simulink model "rev0BB"  (R2017b)
settings: Solver=FixedStepDiscrete  StartTime=0  StopTime=(((preLen+100+dataLenSymbols)*1+pad_first*3)*basePer)  RelTol=1e-3
values from neighbouring files (symbols this model uses):
  ack_stf_len_symbols = length(x_ACK_STF)    [rev0BB_setup.m]
  agc_delay_lag = 32    [rev0BB_setup.m]
  agc_detector_coef = ones(1,agc_detector_taps)./agc_detector_taps    [rev0BB_setup.m]
  agc_on = true    [rev0BB_startup.m]
  agc_sat_low = -agcSaturation    (= -12)    [rev0BB_setup.m]
  agc_sat_up = agcSaturation    (= 12)    [rev0BB_setup.m]
  agcDesired = 0    [rev0BB_setup.m]
  agcExpDomain = agcSaturation    (= 12)    [rev0BB_setup.m]
  agcExpResolution = 2^-5    (= 0.03125)    [rev0BB_setup.m]
  agcPwrAvgNum = 128    [rev0BB_setup.m]
  agcSaturation = 12    [rev0BB_setup.m]
  agcSettleThresh = 0.65    [rev0BB_setup.m]
  agcStep = 2^-8    (= 0.00390625)    [rev0BB_setup.m]
  atanDomain = 5    [rev0BB_setup.m]
  atanDomainTiming = 256    [rev0BB_setup.m]
  atanResolution = 2^-9    (= 0.001953125)    [rev0BB_setup.m]
  atanResolutionTiming = 2^-5    (= 0.03125)    [rev0BB_setup.m]
  averaging_num = ones(1, averaging_samples)    [rev0BB_setup.m]
  averaging_samples = 128    [rev0BB_setup.m]
  awgnSeed = abs(dBSnrRange(dBSnrInd)*1000+trial+10000000)    [plotBer.m]    (also in rev0BB_startup.m = 67)
  basePer = 1/baseFreq    (= 5e-08)    [rev0BB_setup.m]
  bitsPerSymbolHeader = log2(radixHeader)    [rev0BB_setup.m]
  bitsPerSymbolMax = log2(radixMax)    [rev0BB_setup.m]
  cal_sig_i_mult = 1.0    (= 1)    [rev0BB_startup.m]
  cal_sig_i_offset = 0.0    (= 0)    [rev0BB_startup.m]
  cal_sig_q_mult = 1.0    (= 1)    [rev0BB_startup.m]
  cal_sig_q_offset = 0.0    (= 0)    [rev0BB_startup.m]
  cefEarlyWarning = 256    [rev0BB_setup.m]
  cefLen = length(x_CEF)    [rev0BB_setup.m]
  channelFIR = zeros(1, round(maxSampleDelay)+1)    [rev0BB_startup.m]
  coarseCFOAdaptDelay = 1    [rev0BB_setup.m]
  cr_i = 0.020    (= 0.02)    [rev0BB_setup.m]
  cr_i_preamp = 2^-9    (= 0.001953125)    [rev0BB_setup.m]
  cr_int1_sat_low = -cr_integrator1_saturation    (= -0.6)    [rev0BB_setup.m]
  cr_int1_sat_up = cr_integrator1_saturation    (= 0.6)    [rev0BB_setup.m]
  cr_integrator1_decay = 1    [rev0BB_setup.m]
  cr_integrator1_saturation = 0.6    [rev0BB_setup.m]
  cr_mult_pipeline = 0    [rev0BB_setup.m]
  cr_p = 0.015    [rev0BB_setup.m]
  cr_sat2_low = -cr_saturation2    (= -0.6)    [rev0BB_setup.m]
  cr_sat2_up = cr_saturation2    (= 0.6)    [rev0BB_setup.m]
  cr_smooth_num = (1/cr_smooth_samples).*ones(1, cr_smooth_samples)    [rev0BB_setup.m]
  D_128 = [ 1,  8,  2,  4, 16, 32, 64]    [golay.m]    (also in rev0BB_setup.m)
  D_32 = [ 1,  4,  8,  2, 16]    [golay.m]    (also in rev0BB_setup.m)
  dataLenSymbols = header_len_bytes*8/bitsPerSymbolHeader + frame_len_bytes*8/bitsPerSymbol    [rev0BB_setup.m]
  default_channel = 3    [rev0BB_setup.m]
  dmm_coefs = ones(1,dmm_samples)./dmm_samples    [rev0BB_setup.m]
  dst_field_len = 8    [rev0BB_setup.m]
  expDomain = 3.3    [rev0BB_setup.m]
  expResolution = 2^-5    (= 0.03125)    [rev0BB_setup.m]
  expTol = .1    (= 0.1)    [rev0BB_setup.m]
  flush_delay = regular_pipeline*2+mult_pipeline+4    (= 4)    [rev0BB_setup.m]
  frac_lut_domain = 256    [rev0BB_setup.m]
  frac_lut_domain_cr = 64    [rev0BB_setup.m]
  frac_lut_range_max = 512    [rev0BB_setup.m]
  frac_lut_range_max_coarse_cfo = 127    [rev0BB_setup.m]
  frac_lut_range_max_cr = 127    [rev0BB_setup.m]
  frac_lut_range_min = -frac_lut_range_max    (= -512)    [rev0BB_setup.m]
  frac_lut_range_min_coarse_cfo = -frac_lut_range_max_coarse_cfo    (= -127)    [rev0BB_setup.m]
  frac_lut_range_min_cr = -frac_lut_range_max_cr    (= -127)    [rev0BB_setup.m]
  frac_lut_table_breaks = -frac_lut_domain:frac_lut_res:(frac_lut_domain-1)    [rev0BB_setup.m]
  frac_lut_table_breaks_coarse_cfo = -frac_lut_domain_coarse_cfo:frac_lut_res_coarse_cfo:(frac_lut_domain_coarse_cfo-1)    [rev0BB_setup.m]
  frac_lut_table_breaks_cr = -frac_lut_domain_cr:frac_lut_res_cr:(frac_lut_domain_cr-1)    [rev0BB_setup.m]
  frac_lut_table_data = 1./frac_lut_table_breaks    [rev0BB_setup.m]
  frac_lut_table_data_coarse_cfo = 1./frac_lut_table_breaks_coarse_cfo    [rev0BB_setup.m]
  frac_lut_table_data_cr = 1./frac_lut_table_breaks_cr    [rev0BB_setup.m]
  freeze_en_agc = true    [rev0BB_startup.m]
  freeze_en_cr_int1 = false    [rev0BB_startup.m]
  freeze_en_cr_int2 = false    [rev0BB_startup.m]
  freeze_en_cr_phase = false    [rev0BB_startup.m]
  freeze_en_tr_int1 = false    [rev0BB_startup.m]
  freeze_en_tr_int2 = false    [rev0BB_startup.m]
  freeze_en_tr_phase = false    [rev0BB_startup.m]
  freeze_on_cef_done = true    [rev0BB_startup.m]
  freeze_on_stf_done = false    [rev0BB_startup.m]
  freeze_on_valid = true    [rev0BB_startup.m]
  golay_type = 32    [rev0BB_setup.m]
  guardInt = int16(4)    [rev0BB_setup.m]
  guardTol = int16(5)    [rev0BB_setup.m]
  header_len_bytes = 8    [rev0BB_setup.m]
  lineWidth = 60    [rev0BB_setup.m]
  lmsEqDepth = 38    [rev0BB_setup.m]
  lmsStep_init = 0.006    [rev0BB_setup.m]
  lmsStep_meta = (lmsStep_final - lmsStep_init)/cefLen    [rev0BB_setup.m]
  lnDomain = 16    [rev0BB_setup.m]
  lnResolution = 2^-5    (= 0.03125)    [rev0BB_setup.m]
  local_node_id = 2    [rev0BB_startup.m]
  maxMsgSize = length(xSpectrum_PRE)+dataLenSymbols+300    [rev0BB_setup.m]
  minSTFPeaks = 3    [rev0BB_setup.m]
  mod_scheme_len_bytes = 1    [rev0BB_setup.m]
  modBPS = [1, 2, 4]    [rev0BB_setup.m]
  modKeys = [0, 1, 2]    [rev0BB_setup.m]
  mult_pipeline = 0    [rev0BB_setup.m]
  overSampleFreq = 80e6    (= 80000000)    [rev0BB_setup.m]
  overSamplePer = 1/overSampleFreq    (= 1.25e-08)    [rev0BB_setup.m]
  pad_first = 1000    [createTestVectors.m]
  post_cr_i_offset = 0    [rev0BB_startup.m]
  post_cr_q_offset = 0    [rev0BB_startup.m]
  preambleSequentialDetect = 2    [rev0BB_setup.m]
  preLen = length(x_PRE)    [rev0BB_setup.m]
  qam16_demod_scale_factor = qam16_hdl_distance/qam16_power_normalized_distance    [rev0BB_setup.m]
  rcRxFilt = [0.000303163120401141 -0.00118915940834234 -0.00187387637177 -0.00124167532697737 0.00029186889076529 0.00164526160586517 0.00182432050803312 0.000652133621739543 -0.00105668254004908 -0.00204011570659167 -0.00150058088768918 0.00026138356356816 0.0019831869994874 0.00231075800085521 0.000821993419120097 -0.00154687337975486 -0.00305430783933469 -0.00238186490079127 0.000301216962040692 0.00325307 ...(+2001 chars)    [rev0BB_setup.m]
  rcTxFilt = [0.000303163120401141 -0.00118915940834234 -0.00187387637177 -0.00124167532697737 0.00029186889076529 0.00164526160586517 0.00182432050803312 0.000652133621739543 -0.00105668254004908 -0.00204011570659167 -0.00150058088768918 0.00026138356356816 0.0019831869994874 0.00231075800085521 0.000821993419120097 -0.00154687337975486 -0.00305430783933469 -0.00238186490079127 0.000301216962040692 0.00325307 ...(+2001 chars)    [rev0BB_setup.m]
  regular_pipeline = 0    [rev0BB_setup.m]
  rx_gain = 1    [rev0BB_setup.m]
  rx_gain_i = 1    [rev0BB_setup.m]
  rx_gain_q = 1    [rev0BB_setup.m]
  rx_impare_i_offset = 0    [rev0BB_startup.m]
  rx_impare_i_scale = 1    [rev0BB_startup.m]
  rx_impare_q_offset = 0    [rev0BB_startup.m]
  rx_impare_q_scale = 1    [rev0BB_startup.m]
  rx_offset_correction_i = 0    [rev0BB_startup.m]
  rx_offset_correction_q = 0    [rev0BB_startup.m]
  sin_source_amp = 1    [rev0BB_setup.m]
  sin_source_freq = 250e6/16    (= 15625000)    [rev0BB_setup.m]
  slowPer = overSamplePer*slowSample    (= 2.5e-08)    [rev0BB_setup.m]
  std_pkt_type = 0    [rev0BB_setup.m]
  stfLen = length(x_STF)    [rev0BB_setup.m]
  testMsg = cat(1, xCTRL_PRE_adj, header, payload)    [plotBer.m]
  timing_i = 0.25    [rev0BB_setup.m]
  ... (+25 more)
undefined symbols (not defined in the file or in its folder): cr_integrator2_saturation, doppler, i, magnitude, useFadingChannel
libraries: helperLib x128, simulink x90, golayLib x34, dspsigops x32, commfilt2 x27, commdigbbndpm3 x8, hdlsllib x6, dsparch4 x4, commdigbbndam3 x4, commchan3 x2, commrflib2 x2, commcrc2 x2
(part 1 of 10)
settings Model: FPTRunName=FPA_Reference  ExtModeTrigDuration=100  Creator=cyarp  LastModifiedBy=cyarp
settings SolverCC: InsertRTBMode=Always
settings DataIOCC: LimitDataPoints=on  SaveFinalState=on  SaveFormat=StructureWithTime  SaveOutput=off  SaveState=on  StateSaveName=tmp_raccel_xout  SignalLoggingName=tmp_raccel_logsout
settings OptimizationCC: DefaultParameterBehavior=Inlined  UseDivisionForNetSlopeComputation=on  UseFloatMulNetSlope=on  InlineInvariantSignals=on  PassReuseOutputArgsAs=Individual arguments  EfficientFloat2IntCast=on  SimCompilerOptimization=on  OptimizeBlockOrder=speed  DifferentSizesBufferReuse=on
settings DebuggingCC: AlgebraicLoopMsg=error  SolverPrmCheckMsg=warning  SingleTaskRateTransMsg=error  ParameterTunabilityLossMsg=error  SFUnexpectedBacktrackingDiag=warning  SFNoUnconditionalDefaultTransitionDiag=warning  SFExecutionAtInitializationDiag=none
settings HardwareCC: ProdBitPerLong=64  ProdHWDeviceType=Intel->x86-64 (Linux 64)  TargetBitPerLong=64  TargetBitPerPointer=64  TargetBitPerSizeT=64  TargetBitPerPtrDiffT=64  TargetLongLongMode=on  TargetIntDivRoundTo=Zero  TargetEndianess=LittleEndian  TargetWordSize=64  TargetHWDeviceType=MATLAB Host
settings ModelReferenceCC: PropagateSignalLabelsOutOfModel=off
settings SFSimCC: MATLABDynamicMemAlloc=off
settings RTWCC: SystemTargetFile=ert.tlc  TemplateMakefile=ert_default_tmf  GenerateReport=on  SaveLog=on  RTWUseSimCustomCode=on  BuildConfiguration=Faster Runs  IncludeHyperlinkInReport=on  LaunchReport=on  CreateSILPILBlock=SIL  GenerateTraceInfo=on  GenerateTraceReport=on  GenerateTraceReportSl=on  GenerateTraceReportSf=on  GenerateTraceReportEml=on  GenerateCodeMetricsReport=on  GenerateCodeReplacementReport=on
settings CodeAppCC: ForceParamTrailComments=on  IgnoreCustomStorageClasses=off  OperatorAnnotations=on  SimulinkDataObjDesc=on  SFDataObjDesc=on  InsertBlockDesc=on
settings ERTTargetCC: TargetLangStandard=C99 (ISO)  GenerateSampleERTMain=on  ERTCustomFileTemplate=example_file_process.tlc
settings ConfigComp: CovScope=Subsystem  CovPath=receiver  CovMetricSettings=dw  CovHtmlReporting=on  CovSaveCumulativeToWorkspaceVar=on  CovSaveSingleToWorkspaceVar=on  CovExternalEMLEnable=off  CovSFcnEnable=off
settings SimscapeCC: SimscapeNormalizeSystem=off

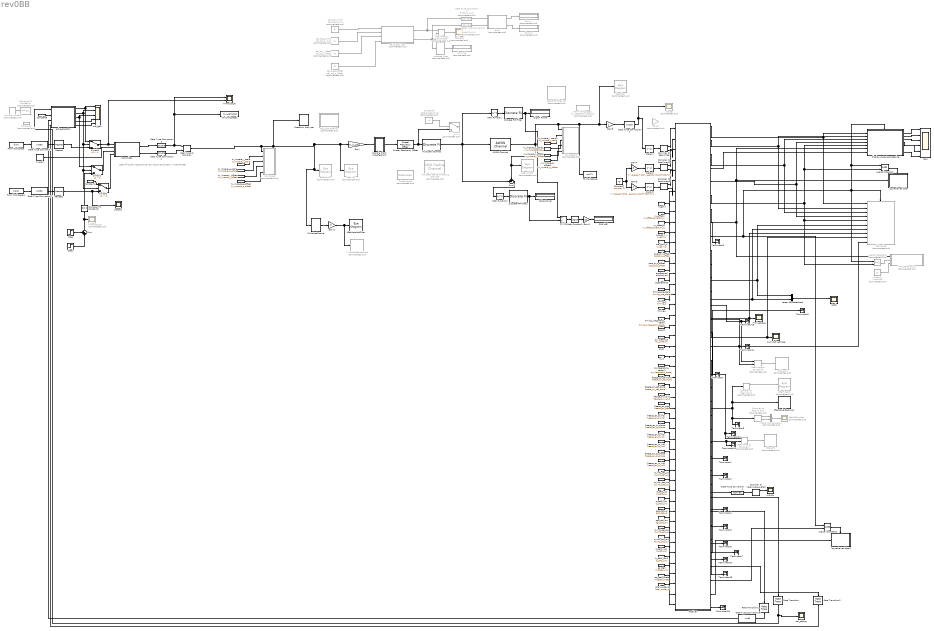
== system rev0BB ==
  note: Zero filling for upsampling now occurs explicitally in transmitter
  " AfterAGC" : ConstellationDiagram  Commented=on
  " AfterCarrierRecovery" : ConstellationDiagram
  ADC_DAC Filtering : Subsystem  Commented=on
  ADC_DAC Filtering1 : Subsystem  Commented=on
  AWGN Channel : commchan3/AWGN Channel  InputProcessing=Columns as channels (frame based)  seed=awgnSeed  noiseMode="Signal to noise ratio  (SNR)"  EbNodB=awgnEbN0  EsNodB=10  SNRdB=awgnSNR  bitsPerSym=1  Ps=1  Tsym=basePer  variance=1
  After AWGN : EyeDiagram  Commented=on
  After LPF : EyeDiagram  Commented=on
  AfterChan : EyeDiagram  Commented=on
  AfterCrSamples : Scope  Commented=on
  AfterFineCR : EyeDiagram  Commented=on
  AfterMatchedFilter : EyeDiagram
  Before LPF : EyeDiagram  Commented=on
  CaCb : Scope  NumInputPorts=3
  CalSignal : Scope  Commented=on
  Compare To Constant1 : simulink/Logic and Bit Operations/Compare To Constant  Commented=on  relop===  const=511  OutDataTypeStr=boolean
  Compare To Constant2 : simulink/Logic and Bit Operations/Compare To Constant  relop===  const=0  OutDataTypeStr=boolean
  Complex to Magnitude-Angle2 : ComplexToMagnitudeAngle
  Complex to Real-Imag : ComplexToRealImag
  Complex to Real-Imag1 : ComplexToRealImag
  Complex to Real-Imag2 : ComplexToRealImag  Commented=on
  Complex to Real-Imag3 : ComplexToRealImag
  Complex to Real-Imag4 : ComplexToRealImag  Commented=on
  Constant : Constant  Commented=on  Value=lineWidth
  Constant2 : Constant  Value=complex(0)  OutDataTypeStr=Inherit: Inherit via back propagation  SampleTime=-1
  Constant3 : Constant  Commented=on  Value=useFadingChannel  OutDataTypeStr=boolean
  Constant4 : Constant  Value=0  OutDataTypeStr=uint32  SampleTime=-1
  Constant5 : Constant  Value=false  OutDataTypeStr=Inherit: Inherit via back propagation  SampleTime=-1
  Constant6 : Constant  Commented=on  Value=5  OutDataTypeStr=Inherit: Inherit via back propagation  SampleTime=-1
  Counter Limited : simulink/Sources/Counter Limited  Commented=on  uplimit=511  tsamp=-1
  CumulativePhase : Scope
  Data Type Conversion : DataTypeConversion  OutDataTypeStr=uint32  RndMeth=Nearest
  Data Type Conversion1 : DataTypeConversion  OutDataTypeStr=single
  Data Type Conversion2 : DataTypeConversion  OutDataTypeStr=double  RndMeth=Nearest
  Data Type Conversion3 : DataTypeConversion  OutDataTypeStr=double  RndMeth=Nearest
  Data Type Conversion4 : DataTypeConversion
  Data Type Conversion5 : DataTypeConversion  Commented=on  OutDataTypeStr=fixdt(1,14,11)
  Data Type Conversion6 : DataTypeConversion  Commented=on  OutDataTypeStr=fixdt(1,14,11)
  Data Type Conversion7 : DataTypeConversion  OutDataTypeStr=uint32  RndMeth=Nearest
  Data Type Conversion9 : DataTypeConversion  OutDataTypeStr=uint8
  Delay1 : Delay  DelayLength=3  InitialCondition=0
  Delay2 : Delay  DelayLength=(preLen+100+dataLenSymbols+100)*4*2  InitialCondition=0
  Delay3 : Delay  DelayLength=(preLen+100+dataLenSymbols+100)*4*1  InitialCondition=0
  Discrete FIR Filter : DiscreteFir  Coefficients=ones(1,10000)./10000  InputProcessing=Columns as channels (frame based)
  Discrete FIR Filter1 : DiscreteFir  Coefficients=ones(1,10000)./10000  InputProcessing=Columns as channels (frame based)
  Divide : Product  Inputs=*/
  FSM : Scope  NumInputPorts=6
  From Workspace : FromWorkspace  VariableName=simX  SampleTime=basePer*1  Interpolate=off  OutputAfterFinalValue=Setting to zero
  From Workspace1 : FromWorkspace  VariableName=modX  SampleTime=basePer*1  Interpolate=off  OutputAfterFinalValue=Setting to zero
  From Workspace2 : FromWorkspace  Commented=on  VariableName=tx_integration_test_sig  SampleTime=overSamplePer*1  Interpolate=off  OutputAfterFinalValue=Setting to zero
  Gain : Gain  Gain=tx_rx_gain
  Gain1 : Gain  Gain=10
  Gain2 : Gain  Gain=.5
  Gain3 : Gain
  Gain4 : Gain  Gain=.5  OutDataTypeStr=Inherit: Same as input
  Gain5 : Gain  Gain=.1  OutDataTypeStr=Inherit: Same as input
  Gain6 : Gain  Commented=on  Gain=.001  OutDataTypeStr=Inherit: Same as input
  IQ_Impare : Subsystem  Commented=on
  IQ_Impare1 : Subsystem  Commented=on
  LMS Err : Scope
  Logical Operator : Logic  AllPortsSameDT=off  OutDataTypeStr=boolean
  Logical Operator1 : Logic  Commented=on  AllPortsSameDT=off  OutDataTypeStr=boolean
  Logical Operator2 : Logic  AllPortsSameDT=off  OutDataTypeStr=boolean
  MATLAB Function : MATLAB Function  Commented=on  TreatAsAtomicUnit=on
  Math Function : Math  Operator=magnitude^2  OutputSignalType=real  SaturateOnIntegerOverflow=on
  Math Function1 : Math  Operator=magnitude^2  OutputSignalType=real  SaturateOnIntegerOverflow=on
  Math Function2 : Math  Operator=log10  OutputSignalType=real  SaturateOnIntegerOverflow=on
  Multipath Channel : DiscreteFir  Coefficients=channelFIR  InputProcessing=Columns as channels (frame based)
  Multipath Rayleigh Fading Channel : commchan3/SISO Fading Channel  Commented=on  PathDelays=chanDelays  AveragePathGains=chanPathGains  NormalizePathGains=on  FadingDistribution=Rayleigh  KFactor=3  DirectPathDopplerShift=0  DirectPathInitialPhase=0  MaximumDopplerShift=maxDopplerHz  DopplerSpectrum=doppler('Flat')  RandomStream=mt19937ar with seed  RandomNumGenerator=shr3cong  Seed=awgnSeed  PathGainsOutputPort=on  ChannelFilterDelayOutputPort=on  SimulateUsing=Interpreted execution  Visualization=Off  PathsForDopplerDisplay=1  SamplesToDisplay=25%
      settings: SourceProductName=Communications System Toolbox
  Noise Power : Display
  Origional : ConstellationDiagram  Commented=on
  Phase Noise : commrflib2/Phase Noise  Commented=on  PhNs=-100  Fo=10000  Fs=overSampleFreq  seed=2137
      settings: SourceProductName=Communications System Toolbox  SourceProductBaseCode=CM
  Phase/ Frequency Offset : commrflib2/Phase// Frequency Offset  phaseOffset=rxPhaseOffset  freqPort=off  freqOffset=freqOffsetHz
      settings: SourceProductName=Communications System Toolbox
  Rate Transition : RateTransition
  Rate Transition1 : RateTransition
  Rate Transition2 : RateTransition
  Real-Imag to Complex : RealImagToComplex
  Real-Imag to Complex2 : RealImagToComplex  Commented=on
  Real-Imag to Complex3 : RealImagToComplex  Commented=on
  Real-Imag to Complex6 : RealImagToComplex  Commented=on
  Repeat : dspsigops/Repeat  N=4  RateOptions=Allow multirate processing  ic=0  mode=Unused parameter value
      settings: SourceProductName=DSP System Toolbox
  Repeat1 : dspsigops/Repeat  N=4  RateOptions=Allow multirate processing  ic=0  mode=Unused parameter value
      settings: SourceProductName=DSP System Toolbox
  RxRaisedCosine : Subsystem
  SNR (dB) : Display
  Sample Clock Imperfections : Subsystem
  Scope : Scope  Commented=on
  Scope1 : Scope
  Signal Power : Display
  Spectrum Analyzer : SpectrumAnalyzer
  Step : Step  Time=(pad_first*basePer)  SampleTime=basePer/4
  Step1 : Step  Time=(pad_first+length(testMsg))*basePer  After=-1  SampleTime=basePer/4
  Sum : Sum  Inputs=++|
  Sum3 : Sum  Inputs=+-|
  Switch : Switch  Commented=on  Criteria=u2 > Threshold
  Switch1 : Switch  Criteria=u2 > Threshold
  Switch2 : Switch  Criteria=u2 > Threshold
  Switch3 : Switch  Criteria=u2 > Threshold
  Terminator{,1..16} (17 alike) : Terminator
  Time Scope : Scope  NumInputPorts=2
  Time Scope1 : Scope  Commented=on
  TimingDelay : Scope
  To Workspace : ToWorkspace  VariableName=rawTx  SampleTime=-1
      settings: Save2DSignal=2-D array (concatenate along first dimension)
  To Workspace1 : ToWorkspace  VariableName=tx_i_samples  SampleTime=-1
      settings: Save2DSignal=2-D array (concatenate along first dimension)
  TxConstAfterMatched : ConstellationDiagram  Commented=on
  Vector Concatenate1 : Concatenate  Commented=on  Mode=Multidimensional array  ConcatenateDimension=2
  Vector Concatenate3 : Concatenate  Mode=Multidimensional array  ConcatenateDimension=2
  ack_debug : Scope
  ack_gen : Scope  NumInputPorts=5
  ack_generator : Subsystem
  agcDesired : Constant  Value=agcDesired  OutDataTypeStr=Inherit: Inherit via back propagation  SampleTime=-1
  agcStepSize : Constant  Value=agcStep  OutDataTypeStr=Inherit: Inherit via back propagation  SampleTime=-1
  agc_on : Constant  Value=agc_on  OutDataTypeStr=Inherit: Inherit via back propagation  SampleTime=-1
  agc_sat_low : Constant  Value=agc_sat_low  OutDataTypeStr=Inherit: Inherit via back propagation  SampleTime=-1
  agc_sat_up : Constant  Value=agc_sat_up  OutDataTypeStr=Inherit: Inherit via back propagation  SampleTime=-1
  average_filter : helperLib/average_filter  Commented=on  pipe=regular_pipeline  samples=128  gain=1/128
  cal_sig_i_mult : Constant  Commented=on  Value=cal_sig_i_mult  OutDataTypeStr=Inherit: Inherit via back propagation  SampleTime=overSamplePer
  cal_sig_i_offset : Constant  Commented=on  Value=cal_sig_i_offset  OutDataTypeStr=Inherit: Inherit via back propagation  SampleTime=overSamplePer
  cal_sig_q_mult : Constant  Commented=on  Value=cal_sig_q_mult  OutDataTypeStr=Inherit: Inherit via back propagation  SampleTime=overSamplePer
  cal_sig_q_offset : Constant  Commented=on  Value=cal_sig_q_offset  OutDataTypeStr=Inherit: Inherit via back propagation  SampleTime=overSamplePer
  cal_signal_gen : Subsystem  Commented=on
  cr_i1 : Constant  Value=cr_i  OutDataTypeStr=Inherit: Inherit via back propagation  SampleTime=-1
  cr_i_preamp1 : Constant  Value=cr_i_preamp  OutDataTypeStr=Inherit: Inherit via back propagation  SampleTime=-1
  cr_int1_sat_low : Constant  Value=cr_int1_sat_low  OutDataTypeStr=Inherit: Inherit via back propagation  SampleTime=-1
  cr_int1_sat_up : Constant  Value=cr_int1_sat_up  OutDataTypeStr=Inherit: Inherit via back propagation  SampleTime=-1
  cr_integrator1_decay1 : Constant  Value=cr_integrator1_decay  OutDataTypeStr=Inherit: Inherit via back propagation  SampleTime=-1
  cr_p1 : Constant  Value=cr_p  OutDataTypeStr=Inherit: Inherit via back propagation  SampleTime=-1
  cr_sat2_low : Constant  Value=cr_sat2_low  OutDataTypeStr=Inherit: Inherit via back propagation  SampleTime=-1
  cr_sat2_up : Constant  Value=cr_sat2_up  OutDataTypeStr=Inherit: Inherit via back propagation  SampleTime=-1
  debug_log : Subsystem  Commented=on
  display_output_processing : Subsystem
  dmm : Subsystem  Commented=on
  dmm I : Display  Commented=on
  dmm Q : Display  Commented=on
  dmm Q1 : Display  Commented=on
  eq_step : Constant  Value=lmsStep_init  OutDataTypeStr=Inherit: Inherit via back propagation  SampleTime=-1
  eq_step_meta : Constant  Value=lmsStep_meta  OutDataTypeStr=Inherit: Inherit via back propagation  SampleTime=-1
  freeze_en_agc : Constant  Value=freeze_en_agc  OutDataTypeStr=Inherit: Inherit via back propagation  SampleTime=-1
  freeze_en_cr_int1 : Constant  Value=freeze_en_cr_int1  OutDataTypeStr=Inherit: Inherit via back propagation  SampleTime=-1
  freeze_en_cr_int2 : Constant  Value=freeze_en_cr_int2  OutDataTypeStr=Inherit: Inherit via back propagation  SampleTime=-1
  freeze_en_cr_phase : Constant  Value=freeze_en_cr_phase  OutDataTypeStr=Inherit: Inherit via back propagation  SampleTime=-1
  freeze_en_tr_int1 : Constant  Value=freeze_en_tr_int1  OutDataTypeStr=Inherit: Inherit via back propagation  SampleTime=-1
  freeze_en_tr_int2 : Constant  Value=freeze_en_tr_int2  OutDataTypeStr=Inherit: Inherit via back propagation  SampleTime=-1
  freeze_en_tr_phase : Constant  Value=freeze_en_tr_phase  OutDataTypeStr=Inherit: Inherit via back propagation  SampleTime=-1
  freeze_on_cef_done : Constant  Value=freeze_on_cef_done  OutDataTypeStr=Inherit: Inherit via back propagation  SampleTime=-1
  freeze_on_stf_done : Constant  Value=freeze_on_stf_done  OutDataTypeStr=Inherit: Inherit via back propagation  SampleTime=-1
  freeze_on_valid : Constant  Value=freeze_on_valid  OutDataTypeStr=Inherit: Inherit via back propagation  SampleTime=-1
  local_node_id : Constant  Value=local_node_id  OutDataTypeStr=Inherit: Inherit via back propagation  SampleTime=-1
  log recieved data : Subsystem
  log recieved data1 : Subsystem
  post_cr_i_offset : Constant  Value=post_cr_i_offset  OutDataTypeStr=fixdt(1,14,11)  SampleTime=-1
  post_cr_q_offset : Constant  Value=post_cr_q_offset  OutDataTypeStr=fixdt(1,14,11)  SampleTime=-1
  pre_gain_i : Constant  Value=rx_gain_i  OutDataTypeStr=Inherit: Inherit via back propagation  SampleTime=overSamplePer
  pre_gain_q : Constant  Value=rx_gain_q  OutDataTypeStr=Inherit: Inherit via back propagation  SampleTime=overSamplePer
  receiver : Subsystem  TreatAsAtomicUnit=on
  rx_gain : Constant  Value=rx_gain  OutDataTypeStr=Inherit: Inherit via back propagation  SampleTime=overSamplePer
  rx_impare_i_offset1 : Constant  Value=rx_impare_i_offset  OutDataTypeStr=Inherit: Inherit via back propagation  SampleTime=overSamplePer
  rx_impare_i_scale1 : Constant  Value=rx_impare_i_scale  OutDataTypeStr=Inherit: Inherit via back propagation  SampleTime=overSamplePer
  rx_impare_q_offset1 : Constant  Value=rx_impare_q_offset  OutDataTypeStr=Inherit: Inherit via back propagation  SampleTime=overSamplePer
  rx_impare_q_scale1 : Constant  Value=rx_impare_q_scale  OutDataTypeStr=Inherit: Inherit via back propagation  SampleTime=overSamplePer
  rx_offset_i : Constant  Value=rx_offset_correction_i  OutDataTypeStr=Inherit: Inherit via back propagation  SampleTime=overSamplePer
  rx_offset_q : Constant  Value=rx_offset_correction_q  OutDataTypeStr=Inherit: Inherit via back propagation  SampleTime=overSamplePer
  timing_i : Constant  Value=timing_i  OutDataTypeStr=Inherit: Inherit via back propagation  SampleTime=-1
  timing_integrator1_decay : Constant  Value=timing_integrator1_decay  OutDataTypeStr=Inherit: Inherit via back propagation  SampleTime=-1
  timing_p : Constant  Value=timing_p  OutDataTypeStr=Inherit: Inherit via back propagation  SampleTime=-1
  timing_pre_scale : Constant  Value=timing_pre_scale  OutDataTypeStr=Inherit: Inherit via back propagation  SampleTime=-1
  tr_int1_sat_low : Constant  Value=tr_int1_sat_low  OutDataTypeStr=Inherit: Inherit via back propagation  SampleTime=-1
  tr_int1_sat_up : Constant  Value=tr_int1_sat_up  OutDataTypeStr=Inherit: Inherit via back propagation  SampleTime=-1
  tr_sat2_low1 : Constant  Value=tr_sat2_low  OutDataTypeStr=Inherit: Inherit via back propagation  SampleTime=-1
  tr_sat2_up1 : Constant  Value=tr_sat2_up  OutDataTypeStr=Inherit: Inherit via back propagation  SampleTime=-1
  transmitter : Subsystem
  tx_gain : Constant  Value=tx_gain  OutDataTypeStr=Inherit: Inherit via back propagation  SampleTime=overSamplePer
  tx_impare_i_offset : Constant  Value=tx_impare_i_offset  OutDataTypeStr=Inherit: Inherit via back propagation  SampleTime=overSamplePer
  tx_impare_i_scale : Constant  Value=tx_impare_i_scale  OutDataTypeStr=Inherit: Inherit via back propagation  SampleTime=overSamplePer
  tx_impare_q_offset : Constant  Value=tx_impare_q_offset  OutDataTypeStr=Inherit: Inherit via back propagation  SampleTime=overSamplePer
  tx_impare_q_scale : Constant  Value=tx_impare_q_scale  OutDataTypeStr=Inherit: Inherit via back propagation  SampleTime=overSamplePer
  wires:
  From Workspace/1 -> Data Type Conversion/1
  Gain/1 -> Sample Clock Imperfections/1(In1)
  receiver/1(stf) -> display_output_processing/1(stf), debug_log/1(stfDone)
  receiver/2(cef) -> display_output_processing/2(cef), debug_log/2(cefDone)
  receiver/3(preambleDone_upsample) -> display_output_processing/3(preamble), debug_log/3(preambleDone)
  receiver/6(valid) -> debug_log/5(valid), Logical Operator1/2, display_output_processing/5(valid_in), Logical Operator/2
  receiver/9(strobe) -> Logical Operator2/1, display_output_processing/Enable, Logical Operator/1, Logical Operator1/1, debug_log/Enable
  receiver/7(symbols) -> log recieved data/1(In1), display_output_processing/6(sym), MATLAB Function/1(symbolIn)
  Constant/1 -> MATLAB Function/3(lineWidth)
  Logical Operator1/1 -> MATLAB Function/2(valid)
  Complex to Real-Imag/1 -> receiver/1(baseband_i)
  Complex to Real-Imag/2 -> receiver/2(baseband_q)
  Data Type Conversion/1 -> Repeat/1
  Vector Concatenate3/1 -> CaCb/1
  receiver/10(ca) -> Vector Concatenate3/1, debug_log/6(ca)
  receiver/11(cb) -> debug_log/7(cb), Vector Concatenate3/2
  receiver/12(timingDelay) -> debug_log/8(timingDelay), TimingDelay/1
  receiver/13(cumulativeCarrierPhase) -> CumulativePhase/1, debug_log/9(carrierPhase)
  rx_gain/1 -> receiver/7(gain)
  pre_gain_i/1 -> receiver/10(pre_gain_i)
  pre_gain_q/1 -> receiver/11(pre_gain_q)
  rx_offset_i/1 -> receiver/8(offset_i)
  rx_offset_q/1 -> receiver/9(offset_q)
  Sum/1 -> Compare To Constant2/1, Time Scope1/1
  Step/1 -> Sum/1
  Step1/1 -> Sum/2
  Sample Clock Imperfections/1(Out1) -> Phase/ Frequency Offset/1
  Math Function/1 -> Discrete FIR Filter/1
  Discrete FIR Filter/1 -> Divide/1, Signal Power/1
  Math Function1/1 -> Discrete FIR Filter1/1
  Discrete FIR Filter1/1 -> Divide/2, Noise Power/1
  Sum3/1 -> Math Function1/1
  Divide/1 -> Math Function2/1
  Math Function2/1 -> Gain1/1
  Gain1/1 -> SNR (dB)/1
  receiver/5(failed) -> display_output_processing/4(failed_in), debug_log/4(failed)
  receiver/17(agcCorrection) -> debug_log/10(agcCorrection)
  Logical Operator/1 -> log recieved data/Enable
  receiver/18(after_cr) -> Terminator8/1, Complex to Real-Imag2/1, Complex to Real-Imag4/1, " AfterCarrierRecovery"/1
  Vector Concatenate1/1 -> AfterCrSamples/1
  Complex to Real-Imag2/1 -> Vector Concatenate1/1
  Complex to Real-Imag2/2 -> Vector Concatenate1/2
  Real-Imag to Complex2/1 -> Origional/1
  receiver/14(rawI) -> Terminator10/1, Real-Imag to Complex2/1
  Real-Imag to Complex3/1 -> " AfterAGC"/1
  receiver/20(after_agc_Q) -> Terminator13/1, Real-Imag to Complex3/2
  receiver/19(after_agc_I) -> Terminator12/1, Real-Imag to Complex3/1
  Data Type Conversion3/1 -> Real-Imag to Complex/1, To Workspace1/1, Time Scope/1
  tx_impare_i_scale/1 -> IQ_Impare/2(i_scale)
  tx_impare_q_scale/1 -> IQ_Impare/3(q_scale)
  tx_impare_i_offset/1 -> IQ_Impare/4(i_offset)
  tx_impare_q_offset/1 -> IQ_Impare/5(q_offset)
  rx_impare_i_scale1/1 -> IQ_Impare1/2(i_scale)
  rx_impare_q_scale1/1 -> IQ_Impare1/3(q_scale)
  rx_impare_i_offset1/1 -> IQ_Impare1/4(i_offset)
  rx_impare_q_offset1/1 -> IQ_Impare1/5(q_offset)
  post_cr_i_offset/1 -> receiver/12(post_cr_i_offset)
  post_cr_q_offset/1 -> receiver/13(post_cr_q_offset)
  agcDesired/1 -> receiver/14(agc_desired)
  agcStepSize/1 -> receiver/15(agc_step_size)
  timing_pre_scale/1 -> receiver/16(timing_pre_scale)
  timing_p/1 -> receiver/17(timing_p)
  timing_i/1 -> receiver/18(timing_i)
  timing_integrator1_decay/1 -> receiver/19(timing_integrator1_decay)
  cr_i_preamp1/1 -> receiver/21(cr_i_preamp)
  cr_p1/1 -> receiver/22(cr_p)
  cr_i1/1 -> receiver/23(cr_i)
  cr_integrator1_decay1/1 -> receiver/24(cr_integrator1_decay)
  agc_on/1 -> receiver/20(agc_on)
  display_output_processing/1(stf_done) -> FSM/1
  display_output_processing/2(cef_done) -> FSM/2
  display_output_processing/3(preamble_done) -> FSM/3
  display_output_processing/4(failed) -> FSM/4
  display_output_processing/5(valid) -> FSM/5
  freeze_on_stf_done/1 -> receiver/25(freeze_on_stfDone)
  freeze_on_cef_done/1 -> receiver/26(freeze_on_cefDone)
  freeze_on_valid/1 -> receiver/27(freeze_on_valid)
  freeze_en_cr_int2/1 -> receiver/32(int2_freeze_en_cr)
  freeze_en_agc/1 -> receiver/28(freeze_en_agc)
  freeze_en_tr_int2/1 -> receiver/29(freeze_en_tr_int2)
  freeze_en_tr_phase/1 -> receiver/30(freeze_en_tr_phase)
  cr_int1_sat_up/1 -> receiver/35(cr_int1_sat_up)
  cr_int1_sat_low/1 -> receiver/36(cr_int1_sat_low)
  cr_sat2_up/1 -> receiver/37(cr_sat2_up)
  cr_sat2_low/1 -> receiver/38(cr_sat2_low)
  agc_sat_up/1 -> receiver/39(agc_sat_up)
  agc_sat_low/1 -> receiver/40(agc_sat_low)
  tr_int1_sat_up/1 -> receiver/41(tr_int1_sat_up)
  tr_int1_sat_low/1 -> receiver/42(tr_int1_sat_low)
  freeze_en_cr_phase/1 -> receiver/33(phase_freeze_en_cr)
  freeze_en_cr_int1/1 -> receiver/34(int1_freeze_en_cr)
  freeze_en_tr_int1/1 -> receiver/31(freeze_en_tr_int1)
  Real-Imag to Complex6/1 -> CalSignal/1
  cal_sig_i_mult/1 -> cal_signal_gen/1(cal_sig_i_mult)
  cal_sig_q_mult/1 -> cal_signal_gen/2(cal_sig_q_mult)
  cal_sig_i_offset/1 -> cal_signal_gen/3(cal_sig_i_offset)
  cal_sig_q_offset/1 -> cal_signal_gen/4(cal_sig_q_offset)
  cal_signal_gen/1(i_out) -> Data Type Conversion5/1, Real-Imag to Complex6/1
  cal_signal_gen/2(q_out) -> average_filter/1, Data Type Conversion6/1, Real-Imag to Complex6/2
  dmm/1(Out_I) -> dmm I/1
  dmm/2(Out_Q) -> dmm Q/1
  Data Type Conversion5/1 -> dmm/1(In_I)
  Data Type Conversion6/1 -> dmm/2(In_Q)
  tr_sat2_low1/1 -> receiver/44(tr_sat2_low)
  tr_sat2_up1/1 -> receiver/43(tr_sat2_up)
  average_filter/1 -> dmm Q1/1
  receiver/16(agcPwrEst) -> Terminator/1
  receiver/21(freeze_slow) -> Terminator1/1
  receiver/22(freeze_fast) -> Terminator2/1
  RxRaisedCosine/1(Out2) -> Gain2/1
  Gain2/1 -> TxConstAfterMatched/1, AfterMatchedFilter/1
  receiver/8(last) -> Terminator3/1
  eq_step/1 -> receiver/45(eq_step)
  Multipath Channel/1 -> Math Function/1, AWGN Channel/1, Sum3/2
  eq_step_meta/1 -> receiver/46(eq_step_meta)
  Complex to Magnitude-Angle2/1 -> LMS Err/1
  Data Type Conversion4/1 -> Complex to Magnitude-Angle2/1
  receiver/23(eq_ff_lms_err) -> Data Type Conversion4/1
  receiver/25(coarse_cfo_correct_steps) -> Terminator5/1
  receiver/24(eq_ff_lms_weights) -> Terminator4/1
  tx_gain/1 -> transmitter/2(gain)
  transmitter/1(baseband_i) -> Data Type Conversion3/1
  transmitter/2(baseband_q) -> Data Type Conversion2/1
  Switch3/1 -> Time Scope/2, transmitter/1(symbol)
  Delay1/1 -> Complex to Real-Imag/1
  Data Type Conversion2/1 -> Real-Imag to Complex/2
  AWGN Channel/1 -> Gain3/1, AfterChan/1, To Workspace/1, IQ_Impare1/1(In), After AWGN/1, Sum3/1
  Complex to Real-Imag1/1 -> receiver/3(baseband_i1)
  Complex to Real-Imag1/2 -> receiver/4(baseband_q1)
  Delay2/1 -> Complex to Real-Imag1/1
  Complex to Real-Imag3/1 -> receiver/5(baseband_i2)
  Complex to Real-Imag3/2 -> receiver/6(baseband_q2)
  Delay3/1 -> Complex to Real-Imag3/1
  Data Type Conversion1/1 -> Delay1/1, Scope/1
  Gain5/1 -> Delay3/1
  Gain4/1 -> Delay2/1
  Data Type Conversion7/1 -> Repeat1/1
  From Workspace1/1 -> Data Type Conversion7/1
  Switch2/1 -> transmitter/4(ModMode)
  Constant2/1 -> Gain4/1, Gain5/1
  Phase/ Frequency Offset/1 -> Multipath Channel/1, Switch/3
  Constant3/1 -> Switch/2
  Switch1/1 -> transmitter/3(zero)
  ack_generator/2(valid_out) -> Switch3/2, Switch2/2, Switch1/2, ack_gen/2
  Constant4/1 -> Switch2/1
  ack_generator/3(tail_out) -> Switch1/1, ack_gen/3
  Repeat/1 -> Switch3/3
  ack_generator/1(data_out) -> ack_gen/1, Switch3/1
  Constant5/1 -> ack_generator/2(cancel)
  Counter Limited/1 -> Compare To Constant1/1
  ack_generator/4(ack_last) -> ack_gen/4
  Compare To Constant2/1 -> Switch1/3
  receiver/27(crc_err) -> Terminator7/1
  receiver/26(crc_decision) -> Terminator6/1
  local_node_id/1 -> receiver/47(local_node_id)
  receiver/28(ack_this) -> Rate Transition/1
  Data Type Conversion9/1 -> ack_generator/3(dst_in)
  receiver/29(ack_dst) -> Rate Transition1/1
  Rate Transition1/1 -> Data Type Conversion9/1
  Rate Transition/1 -> ack_debug/1, ack_generator/1(ack)
  display_output_processing/7(ack) -> FSM/6
  receiver/4(ack) -> display_output_processing/7(ack_in)
  receiver/32(ack_trigger) -> Terminator9/1
  Rate Transition2/1 -> ack_generator/4(ack_chan)
  ack_generator/5(tx_chan) -> ack_gen/5
  receiver/33(rx_channel) -> Rate Transition2/1
  Complex to Real-Imag4/1 -> AfterFineCR/1
  receiver/15(rawQ) -> Terminator11/1, Real-Imag to Complex2/2
  receiver/30(ack_rx_done) -> Terminator14/1
  receiver/31(ack_rx_dst) -> Terminator15/1
  Repeat1/1 -> Scope1/1, Switch2/3
  Logical Operator2/1 -> log recieved data1/Enable
  receiver/35(packed_symbol) -> log recieved data1/1(In1)
  receiver/34(packed_valid) -> Logical Operator2/2
  receiver/36(packed_last) -> Terminator16/1
  Gain3/1 -> Data Type Conversion1/1
  Real-Imag to Complex/1 -> Spectrum Analyzer/1, After LPF/1, Gain/1, RxRaisedCosine/1(In2), Before LPF/1, IQ_Impare/1(In)

== system rev0BB/ADC_DAC Filtering ==
  In1 : Inport
  Digital AntiAlias : dsparch4/Digital Filter Design  mwdsp_browser_bugfix_var=off
  Digital DC Block : dsparch4/Digital Filter Design  Commented=on  mwdsp_browser_bugfix_var=off
  Out1 : Outport
  wires:
  Digital AntiAlias/1 -> Out1/1
  In1/1 -> Digital AntiAlias/1, Digital DC Block/1

== system rev0BB/ADC_DAC Filtering1 ==
  In1 : Inport
  Digital AntiAlias : dsparch4/Digital Filter Design  mwdsp_browser_bugfix_var=off
  Digital DC Block : dsparch4/Digital Filter Design  Commented=on  mwdsp_browser_bugfix_var=off
  Out1 : Outport
  wires:
  Digital AntiAlias/1 -> Out1/1
  In1/1 -> Digital AntiAlias/1, Digital DC Block/1

== system rev0BB/IQ_Impare ==
  In : Inport
  i_scale : Inport  Port=2
  q_scale : Inport  Port=3
  i_offset : Inport  Port=4
  q_offset : Inport  Port=5
  Add : Sum
  Add1 : Sum
  Complex to Real-Imag3 : ComplexToRealImag
  Product2 : Product
  Product3 : Product
  Real-Imag to Complex : RealImagToComplex
  Out : Outport
  wires:
  Add/1 -> Real-Imag to Complex/1
  Complex to Real-Imag3/2 -> Product3/1
  Complex to Real-Imag3/1 -> Product2/1
  Add1/1 -> Real-Imag to Complex/2
  q_scale/1 -> Product3/2
  In/1 -> Complex to Real-Imag3/1
  Real-Imag to Complex/1 -> Out/1
  q_offset/1 -> Add1/2
  i_scale/1 -> Product2/2
  i_offset/1 -> Add/2
  Product2/1 -> Add/1
  Product3/1 -> Add1/1

== system rev0BB/IQ_Impare1 ==
  In : Inport
  i_scale : Inport  Port=2
  q_scale : Inport  Port=3
  i_offset : Inport  Port=4
  q_offset : Inport  Port=5
  Add : Sum
  Add1 : Sum
  Complex to Real-Imag3 : ComplexToRealImag
  Product2 : Product
  Product3 : Product
  Real-Imag to Complex : RealImagToComplex
  Out : Outport
  wires:
  Add/1 -> Real-Imag to Complex/1
  Complex to Real-Imag3/2 -> Product3/1
  Complex to Real-Imag3/1 -> Product2/1
  Add1/1 -> Real-Imag to Complex/2
  q_scale/1 -> Product3/2
  In/1 -> Complex to Real-Imag3/1
  Real-Imag to Complex/1 -> Out/1
  q_offset/1 -> Add1/2
  i_scale/1 -> Product2/2
  i_offset/1 -> Add/2
  Product2/1 -> Add/1
  Product3/1 -> Add1/1

== system rev0BB/RxRaisedCosine ==
  In2 : Inport
  Discrete FIR Filter : DiscreteFir  FilterStructure=Direct form transposed  Coefficients=rcRxFilt  AccumDataTypeStr=Inherit: Same as product output
  Out2 : Outport
  wires:
  Discrete FIR Filter/1 -> Out2/1
  In2/1 -> Discrete FIR Filter/1

== system rev0BB/Sample Clock Imperfections ==
  In1 : Inport
  Constant : Constant  Value=txTimingOffset
  Delay : Delay  DelayLength=1  InitialCondition=500+txTimingPhase
  SampleClockDelay : Scope
  Sum : Sum  Inputs=|++
  Variable Fractional Delay : dspsigops/Variable Fractional Delay  mode=OBSOLETE  modeActive=Farrow  dmax=1000  InputProcessing=Columns as channels (frame based)  L=4  FarrowL=4  R=10  alpha=1  ic=0  fallbackFIR=Clip to the minimum value necessary for centered kernel  fallbackFarrow=Clip to the minimum value necessary for centered kernel  noDFT=off  roundingMode=Zero  overflowMode=off
      settings: SourceProductName=DSP System Toolbox  SourceProductBaseCode=DS
  Out1 : Outport
  wires:
  In1/1 -> Variable Fractional Delay/1
  Variable Fractional Delay/1 -> Out1/1
  Constant/1 -> Sum/1
  Sum/1 -> Delay/1
  Delay/1 -> Sum/2, SampleClockDelay/1, Variable Fractional Delay/2

== system rev0BB/ack_generator ==
  ack : Inport  OutDataTypeStr=boolean  SampleTime=basePer
  cancel : Inport  Port=2  OutDataTypeStr=boolean  SampleTime=basePer
  dst_in : Inport  Port=3  OutDataTypeStr=uint8  SampleTime=basePer
  ack_chan : Inport  Port=4  OutDataTypeStr=uint8  SampleTime=basePer
  Delay{,1..8} (9 alike) : Delay  DelayLength=1  InitialCondition=0
  Repeat{1..5} (5 alike) : dspsigops/Repeat  N=4  RateOptions=Allow multirate processing  ic=0  mode=Unused parameter value
      settings: SourceProductName=DSP System Toolbox
  ack_generator : Stateflow chart  TreatAsAtomicUnit=on
  data_out : Outport  SampleTime=overSamplePer
  valid_out : Outport  Port=2  SampleTime=overSamplePer
  tail_out : Outport  Port=3  SampleTime=overSamplePer
  ack_last : Outport  Port=4  SampleTime=overSamplePer
  tx_chan : Outport  Port=5  SampleTime=overSamplePer
  wires:
  ack/1 -> Delay/1
  cancel/1 -> Delay1/1
  Delay4/1 -> Repeat1/1
  Repeat2/1 -> data_out/1
  Delay3/1 -> Repeat2/1
  Repeat1/1 -> valid_out/1
  dst_in/1 -> Delay2/1
  Repeat3/1 -> tail_out/1
  Delay5/1 -> Repeat3/1
  Repeat4/1 -> ack_last/1
  Delay6/1 -> Repeat4/1
  Delay/1 -> ack_generator/1(ack)
  Delay1/1 -> ack_generator/2(cancel)
  Delay2/1 -> ack_generator/3(dst_in)
  ack_generator/1(data_out) -> Delay3/1
  ack_generator/2(valid_out) -> Delay4/1
  ack_generator/3(tail) -> Delay5/1
  ack_generator/4(last) -> Delay6/1
  ack_chan/1 -> Delay7/1
  Delay7/1 -> ack_generator/4(ack_chan)
  Repeat5/1 -> tx_chan/1
  ack_generator/5(tx_chan) -> Delay8/1
  Delay8/1 -> Repeat5/1

== system rev0BB/cal_signal_gen ==
  cal_sig_i_mult : Inport
  cal_sig_q_mult : Inport  Port=2
  cal_sig_i_offset : Inport  Port=3
  cal_sig_q_offset : Inport  Port=4
  Complex to Real-Imag1 : ComplexToRealImag
  Sine Wave : dspsrcs4/Sine Wave  Amplitude=sin_source_amp  Frequency=sin_source_freq  Phase=0  SampleMode=Discrete  OutComplex=Complex  CompMethod=Table lookup  TableSize=Speed  SampleTime=overSamplePer  SamplesPerFrame=1  ResetState=Restart at time zero  OutputFrames=off  dataType=Fixed-point  wordLen=16  udDataType=sfix(16)  fracBitsMode=User-defined  numFracBits=14  OutDataTypeStr=fixdt(1,16,14)  LastOutDataTypeStr=fixdt(1,16,14)
  Sum1 : Sum  Inputs=|++  OutDataTypeStr=Inherit: Inherit via back propagation
  Sum2 : Sum  Inputs=|++  OutDataTypeStr=Inherit: Inherit via back propagation
  pipeline_delay{,1..5} (6 alike) : Delay  DelayLength=regular_pipeline
  pipelined_mult : helperLib/pipelined_mult  d=mult_pipeline*2
  pipelined_mult1 : helperLib/pipelined_mult  d=mult_pipeline*2
  i_out : Outport
  q_out : Outport  Port=2
  wires:
  pipelined_mult/1 -> pipeline_delay5/1
  pipeline_delay1/1 -> q_out/1
  pipeline_delay/1 -> i_out/1
  pipelined_mult1/1 -> pipeline_delay4/1
  Complex to Real-Imag1/2 -> pipelined_mult1/1
  Sum1/1 -> pipeline_delay/1
  Sum2/1 -> pipeline_delay1/1
  cal_sig_i_offset/1 -> pipeline_delay2/1
  cal_sig_q_offset/1 -> pipeline_delay3/1
  Complex to Real-Imag1/1 -> pipelined_mult/1
  cal_sig_i_mult/1 -> pipelined_mult/2
  Sine Wave/1 -> Complex to Real-Imag1/1
  cal_sig_q_mult/1 -> pipelined_mult1/2
  pipeline_delay2/1 -> Sum1/2
  pipeline_delay3/1 -> Sum2/2
  pipeline_delay4/1 -> Sum2/1
  pipeline_delay5/1 -> Sum1/1

== system rev0BB/debug_log ==
  stfDone : Inport
  cefDone : Inport  Port=2
  preambleDone : Inport  Port=3
  failed : Inport  Port=4
  valid : Inport  Port=5
  ca : Inport  Port=6
  cb : Inport  Port=7
  timingDelay : Inport  Port=8
  carrierPhase : Inport  Port=9
  agcCorrection : Inport  Port=10
  Enable : EnablePort
  To Workspace1 : ToWorkspace  VariableName=rx_stfDone  SampleTime=-1
      settings: Save2DSignal=2-D array (concatenate along first dimension)
  To Workspace10 : ToWorkspace  VariableName=rx_agcCorrection  SampleTime=-1
      settings: Save2DSignal=2-D array (concatenate along first dimension)
  To Workspace2 : ToWorkspace  VariableName=rx_cefDone1  SampleTime=-1
      settings: Save2DSignal=2-D array (concatenate along first dimension)
  To Workspace3 : ToWorkspace  VariableName=rx_preambleDone  SampleTime=-1
      settings: Save2DSignal=2-D array (concatenate along first dimension)
  To Workspace4 : ToWorkspace  VariableName=rx_failed  SampleTime=-1
      settings: Save2DSignal=2-D array (concatenate along first dimension)
  To Workspace5 : ToWorkspace  VariableName=rx_valid  SampleTime=-1
      settings: Save2DSignal=2-D array (concatenate along first dimension)
  To Workspace6 : ToWorkspace  VariableName=rx_ca  SampleTime=-1
      settings: Save2DSignal=2-D array (concatenate along first dimension)
  To Workspace7 : ToWorkspace  VariableName=rx_cb  SampleTime=-1
      settings: Save2DSignal=2-D array (concatenate along first dimension)
  To Workspace8 : ToWorkspace  VariableName=rx_timingDelay  SampleTime=-1
      settings: Save2DSignal=2-D array (concatenate along first dimension)
  To Workspace9 : ToWorkspace  VariableName=rx_carrierPhase  SampleTime=-1
      settings: Save2DSignal=2-D array (concatenate along first dimension)
  wires:
  ca/1 -> To Workspace6/1
  cb/1 -> To Workspace7/1
  stfDone/1 -> To Workspace1/1
  carrierPhase/1 -> To Workspace9/1
  agcCorrection/1 -> To Workspace10/1
  valid/1 -> To Workspace5/1
  cefDone/1 -> To Workspace2/1
  timingDelay/1 -> To Workspace8/1
  failed/1 -> To Workspace4/1
  preambleDone/1 -> To Workspace3/1

== system rev0BB/display_output_processing ==
  stf : Inport
  cef : Inport  Port=2
  preamble : Inport  Port=3
  failed_in : Inport  Port=4
  valid_in : Inport  Port=5
  sym : Inport  Port=6
  ack_in : Inport  Port=7
  Enable : EnablePort
  ack_upsample : DataTypeConversion
  cefDone : DataTypeConversion
  failed_ : DataTypeConversion
  preambleDone_upsample : DataTypeConversion
  stfDone : DataTypeConversion
  valid_upsample : DataTypeConversion
  stf_done : Outport
  cef_done : Outport  Port=2
  preamble_done : Outport  Port=3
  failed : Outport  Port=4
  valid : Outport  Port=5
  symbols : Outport  Port=6
  ack : Outport  Port=7
  wires:
  stfDone/1 -> stf_done/1  "stf_done"
  cefDone/1 -> cef_done/1  "cef_done"
  preambleDone_upsample/1 -> preamble_done/1  "preamble_done"
  failed_/1 -> failed/1  "failed_a"
  stf/1 -> stfDone/1
  cef/1 -> cefDone/1
  preamble/1 -> preambleDone_upsample/1
  failed_in/1 -> failed_/1
  valid_upsample/1 -> valid/1  "valid"
  valid_in/1 -> valid_upsample/1
  sym/1 -> symbols/1
  ack_upsample/1 -> ack/1  "valid"
  ack_in/1 -> ack_upsample/1

== system rev0BB/dmm ==
  In_I : Inport
  In_Q : Inport  Port=2
  Discrete FIR Filter : DiscreteFir  FilterStructure=Direct form transposed  Coefficients=dmm_coefs  RndMeth=Round  OutDataTypeStr=Inherit: Same as input
  Discrete FIR Filter1 : DiscreteFir  FilterStructure=Direct form transposed  Coefficients=dmm_coefs  RndMeth=Round  OutDataTypeStr=Inherit: Same as input
  pipeline_delay{1..4} (4 alike) : Delay  DelayLength=regular_pipeline
  Out_I : Outport
  Out_Q : Outport  Port=2
  wires:
  Discrete FIR Filter/1 -> pipeline_delay3/1
  In_I/1 -> pipeline_delay1/1
  Discrete FIR Filter1/1 -> pipeline_delay4/1
  In_Q/1 -> pipeline_delay2/1
  pipeline_delay1/1 -> Discrete FIR Filter/1
  pipeline_delay2/1 -> Discrete FIR Filter1/1
  pipeline_delay3/1 -> Out_I/1
  pipeline_delay4/1 -> Out_Q/1

== system rev0BB/log recieved data ==
  In1 : Inport
  Enable : EnablePort
  To Workspace1 : ToWorkspace  VariableName=data_recieved  SampleTime=-1
      settings: Save2DSignal=2-D array (concatenate along first dimension)
  wires:
  In1/1 -> To Workspace1/1

== system rev0BB/log recieved data1 ==
  In1 : Inport
  Enable : EnablePort
  To Workspace1 : ToWorkspace  VariableName=data_recieved_packed  SampleTime=-1
      settings: Save2DSignal=2-D array (concatenate along first dimension)
  wires:
  In1/1 -> To Workspace1/1
